simulink model "Chapter7Dyn2dCrankRocker"  (Simulink 7.8)
settings: Solver=ode45  StartTime=0.0  StopTime=10.0  RelTol=1e-3
model workspace: external: MAT-File C:\Users\john\Dropbox\Simulation\simulink\Chapter7Dyn2dCrankRocker-SIMULINKPARAM.mat (data not in the file)
values from neighbouring files (symbols this model uses):
  sysmodel =     [AUTO2-SIMULINKPARAM.mat]    (also in AUTO4-SIMULINKPARAM.mat; Chapter7Dyn2dCrankRocker-SIMULINKPARAM.mat; Spatial4barDyn-SIMULINKPARAM.mat)
undefined symbols (not defined in the file or in its folder): selectnum
libraries: MotionSimPlanarLibrary x1
settings Model: Creator=john  LastModifiedBy=john

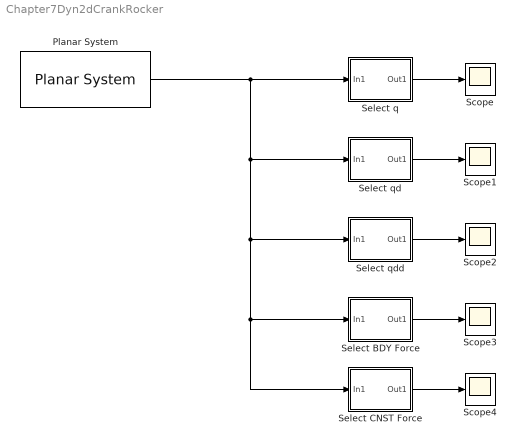
== system Chapter7Dyn2dCrankRocker ==
  Planar System : MotionSimPlanarLibrary/Planar System
  Scope{,1..4} (5 alike) : Scope
      Scope2 settings: SaveName=ScopeData2
      Scope3 settings: SaveName=ScopeData3
      Scope4 settings: SaveName=ScopeData4
  Select BDY Force : Subsystem  AncestorBlock=MotionSimPlanarLibrary/Select BDY Force  mask{Bodynum=3, Selectnum=Fx}
      mask prompts: Bodynum "Body Number"; Selectnum "Select Coordinate"
      mask StyleString: edit,popup(Fx|Fy|Tz)
      mask Display:
      | port_label('input',1,'coord');
      | port_label('output',1,'Fn');
  Select CNST Force : Subsystem  AncestorBlock=MotionSimPlanarLibrary/Select CNST Force  mask{Bodynum=2, Selectnum=Fx}
      mask prompts: Bodynum "Body Number"; Selectnum "Select Coordinate"
      mask StyleString: edit,popup(Fx|Fy|Tz)
      mask Display:
      | port_label('input',1,'coord');
      | port_label('output',1,'Fn');
  Select q : Subsystem  AncestorBlock=MotionSimPlanarLibrary/Select q  mask{Bodynum=2, Selectnum=X}
      mask prompts: Bodynum "Body Number"; Selectnum "Select Coordinate"
      mask StyleString: edit,popup(X|Y|PHI)
      mask Display:
      | port_label('input',1,'coord');
      | port_label('output',1,'q');
  Select qd : Subsystem  AncestorBlock=MotionSimPlanarLibrary/Select qd  mask{Bodynum=2, Selectnum=Xd}
      mask prompts: Bodynum "Body Number"; Selectnum "Select Coordinate"
      mask StyleString: edit,popup(Xd|Yd|PHId)
      mask Display:
      | port_label('input',1,'coord');
      | port_label('output',1,'qd');
  Select qdd : Subsystem  AncestorBlock=MotionSimPlanarLibrary/Select qdd  mask{Bodynum=2, Selectnum=Xdd}
      mask prompts: Bodynum "Body Number"; Selectnum "Select Coordinate"
      mask StyleString: edit,popup(Xdd|Ydd|PHIdd)
      mask Display:
      | port_label('input',1,'coord');
      | port_label('output',1,'qdd');
  wires:
  Planar System/1 -> Select q/1(In1), Select qd/1(In1), Select qdd/1(In1), Select BDY Force/1(In1), Select CNST Force/1(In1)
  Select q/1(Out1) -> Scope/1
  Select qd/1(Out1) -> Scope1/1
  Select qdd/1(Out1) -> Scope2/1
  Select BDY Force/1(Out1) -> Scope3/1
  Select CNST Force/1(Out1) -> Scope4/1

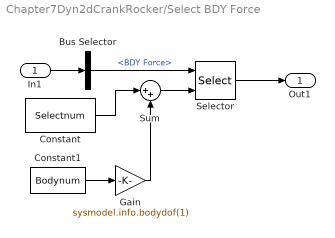
== system Chapter7Dyn2dCrankRocker/Select BDY Force ==
  In1 : Inport
  Bus Selector : BusSelector  OutputSignals=BDY Force
  Constant : Constant  Value=Selectnum
  Constant1 : Constant  Value=Bodynum
  Gain : Gain  Gain=sysmodel.info.bodydof(1)
  Selector : Selector  InputPortWidth=sysmodel.info.bodies*sysmodel.info.bodydof(1)  IndexOptions=Index vector (port)  Indices=[Bodynum+selectnum]  OutputSizes=1
  Sum : Sum  Inputs=|++
  Out1 : Outport
  wires:
  Selector/1 -> Out1/1
  Constant1/1 -> Gain/1
  Sum/1 -> Selector/2
  Constant/1 -> Sum/1
  Gain/1 -> Sum/2
  In1/1 -> Bus Selector/1
  Bus Selector/1 -> Selector/1  "<BDY Force>"

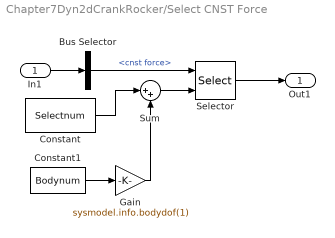
== system Chapter7Dyn2dCrankRocker/Select CNST Force ==
  In1 : Inport
  Bus Selector : BusSelector  OutputSignals=cnst force
  Constant : Constant  Value=Selectnum
  Constant1 : Constant  Value=Bodynum
  Gain : Gain  Gain=sysmodel.info.bodydof(1)
  Selector : Selector  InputPortWidth=sysmodel.info.bodies*sysmodel.info.bodydof(1)  IndexOptions=Index vector (port)  Indices=[Bodynum+selectnum]  OutputSizes=1
  Sum : Sum  Inputs=|++
  Out1 : Outport
  wires:
  Selector/1 -> Out1/1
  Constant1/1 -> Gain/1
  Sum/1 -> Selector/2
  Constant/1 -> Sum/1
  Gain/1 -> Sum/2
  In1/1 -> Bus Selector/1
  Bus Selector/1 -> Selector/1  "<cnst force>"

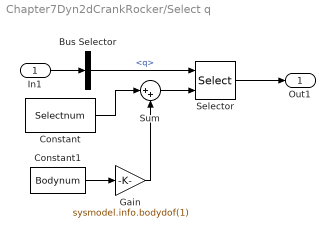
== system Chapter7Dyn2dCrankRocker/Select q ==
  In1 : Inport
  Bus Selector : BusSelector  OutputSignals=q
  Constant : Constant  Value=Selectnum
  Constant1 : Constant  Value=Bodynum
  Gain : Gain  Gain=sysmodel.info.bodydof(1)
  Selector : Selector  InputPortWidth=sysmodel.info.bodies*sysmodel.info.bodydof(1)  IndexOptions=Index vector (port)  Indices=[Bodynum+selectnum]  OutputSizes=1
  Sum : Sum  Inputs=|++
  Out1 : Outport
  wires:
  Selector/1 -> Out1/1
  Constant1/1 -> Gain/1
  Sum/1 -> Selector/2
  Constant/1 -> Sum/1
  Gain/1 -> Sum/2
  In1/1 -> Bus Selector/1
  Bus Selector/1 -> Selector/1  "<q>"

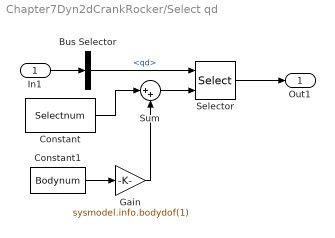
== system Chapter7Dyn2dCrankRocker/Select qd ==
  In1 : Inport
  Bus Selector : BusSelector  OutputSignals=qd
  Constant : Constant  Value=Selectnum
  Constant1 : Constant  Value=Bodynum
  Gain : Gain  Gain=sysmodel.info.bodydof(1)
  Selector : Selector  InputPortWidth=sysmodel.info.bodies*sysmodel.info.bodydof(1)  IndexOptions=Index vector (port)  Indices=[Bodynum+selectnum]  OutputSizes=1
  Sum : Sum  Inputs=|++
  Out1 : Outport
  wires:
  Selector/1 -> Out1/1
  Constant1/1 -> Gain/1
  Sum/1 -> Selector/2
  Constant/1 -> Sum/1
  Gain/1 -> Sum/2
  In1/1 -> Bus Selector/1
  Bus Selector/1 -> Selector/1  "<qd>"

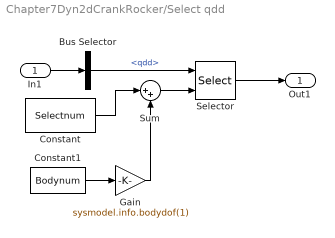
== system Chapter7Dyn2dCrankRocker/Select qdd ==
  In1 : Inport
  Bus Selector : BusSelector  OutputSignals=qdd
  Constant : Constant  Value=Selectnum
  Constant1 : Constant  Value=Bodynum
  Gain : Gain  Gain=sysmodel.info.bodydof(1)
  Selector : Selector  InputPortWidth=sysmodel.info.bodies*sysmodel.info.bodydof(1)  IndexOptions=Index vector (port)  Indices=[Bodynum+selectnum]  OutputSizes=1
  Sum : Sum  Inputs=|++
  Out1 : Outport
  wires:
  Selector/1 -> Out1/1
  Constant1/1 -> Gain/1
  Sum/1 -> Selector/2
  Constant/1 -> Sum/1
  Gain/1 -> Sum/2
  In1/1 -> Bus Selector/1
  Bus Selector/1 -> Selector/1  "<qdd>"
